simulink library "fc_vt_lib"  (Simulink 4.00)
undefined symbols (not defined in the file or in its folder): amb_tmp, compressor_mass_flow_map, compressor_pressure_map, compressor_temperature_rise_map, fc_air_comp_scale, fc_allowable_temp_rise, fc_cathode_pressure_drop, fc_cell_area, fc_cell_num, fc_comp_adeff_max, fc_comp_elec_eff, fc_comp_max_tmp, fc_comp_slpm_air_max, fc_comp_spd_max, fc_comp_voleff_max, fc_condenser_fan_flowrate, fc_condenser_fan_num, fc_condenser_fan_pwr_map, fc_condenser_frontal_area, fc_condenser_scale, fc_coolant_pump_flow_map, fc_coolant_pump_pwr_map, fc_cp_air, fc_cp_h2o_l, fc_cp_stack, fc_fuel_lhv, fc_k_air, fc_max_cathode_inlet_pressure, fc_min_cathode_inlet_pressure, fc_min_cell_volts, fc_min_sys_pwr_req, fc_min_temp_for_heat_rejection, fc_mw_air, fc_mw_h2, fc_mw_h20, fc_o2_percent, fc_p_amb, fc_polar_param_concentration, fc_polar_param_ohmic, fc_polar_param_ohmic_temp, fc_polar_param_ref_temp, fc_polar_param_tafel, fc_polar_param_temperature, fc_polar_param_voc, fc_radiator_bypass_delta_t, fc_radiator_fan_flowrate, fc_radiator_fan_num, fc_radiator_fan_pwr_map, fc_radiator_frontal_area, fc_radiator_no_fan_flowrate, fc_radiator_scale, fc_radiator_spd_ratio_fan_off, fc_radiator_spd_ratio_fan_on, fc_radiator_veh_spd_map, fc_reference_temperature, fc_rh_amb, fc_stack_i_map, fc_stack_pres_cor_map, fc_stack_pres_map, fc_stack_stoich_air_map ... (+10)
libraries: fc_vt_lib x54, simulink3 x9
(part 3 of 3)

== system fc_vt_lib/Main Loop/ambient pressure, temperature & density calc (atm) ==
  note: Ambient
      | temperature [K]
  elevation : Inport  Port=1  LatchInput=off
  Constant1 : Constant  Value=288.15
  Constant2 : Constant  Value=288.15
  Constant3 : Constant  Value=0.0065
  Math Function2 : Math  Operator=pow  OutputSignalType=auto
  Pressure [mbar] : Product  Inputs=*/  Multiplication=Element-wise(.*)  SaturateOnIntegerOverflow=on
  Pressure1 : Constant  Value=-5.255877
  Pressure2 : Constant  Value=0.3483677
  Pressure5 : Constant  Value=1013.25
  Pressure6 : Constant  Value=1013.25
  Product : Product  Inputs=2  Multiplication=Element-wise(.*)  SaturateOnIntegerOverflow=on
  Product2 : Product  Inputs=*/  Multiplication=Element-wise(.*)  SaturateOnIntegerOverflow=on
  Product3 : Product  Inputs=2  Multiplication=Element-wise(.*)  SaturateOnIntegerOverflow=on
  Product5 : Product  Inputs=*/  Multiplication=Element-wise(.*)  SaturateOnIntegerOverflow=on
  Product6 : Product  Inputs=2  Multiplication=Element-wise(.*)  SaturateOnIntegerOverflow=on
  Sum1 : Sum  Inputs=-+  SaturateOnIntegerOverflow=on
  "Ambient pressure [atm] " : Outport  Port=1
  Air density [kg/m3] : Outport  Port=2
  wires:
  Constant1/1 -> Sum1/2
  Pressure2/1 -> Product3/1
  elevation/1 -> Product/1
  Constant3/1 -> Product/2
  Product/1 -> Sum1/1
  Sum1/1 -> Product5/2, Product2/2
  Constant2/1 -> Product5/1
  Product5/1 -> Math Function2/1
  Pressure1/1 -> Math Function2/2
  Math Function2/1 -> Product6/1
  Pressure5/1 -> Product6/2
  Product6/1 -> Pressure [mbar]/1
  Pressure6/1 -> Pressure [mbar]/2
  Pressure [mbar]/1 -> "Ambient pressure [atm] "/1, Product2/1
  Product2/1 -> Product3/2
  Product3/1 -> Air density [kg/m3]/1

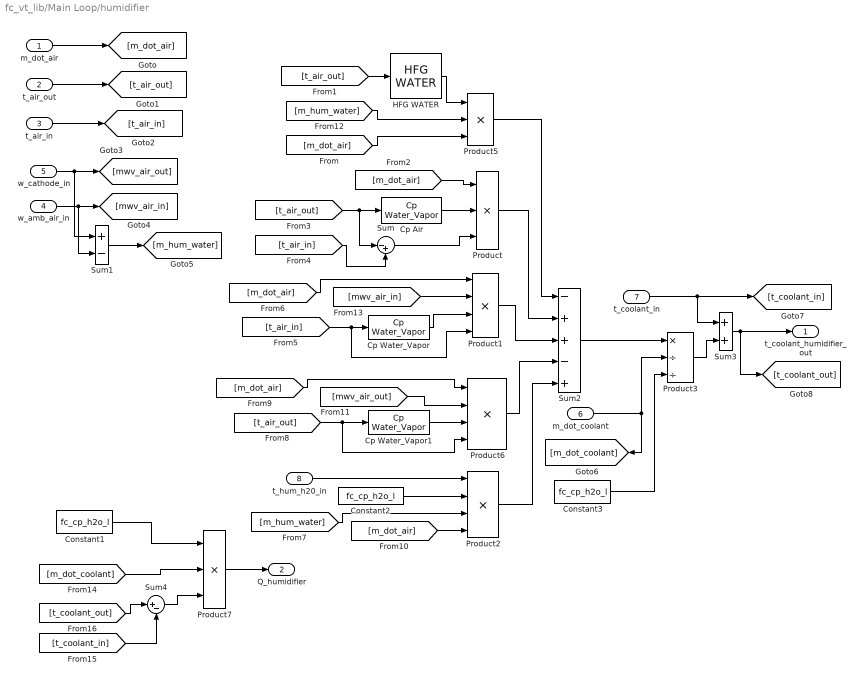
== system fc_vt_lib/Main Loop/humidifier ==
  m_dot_air : Inport  Port=1  LatchInput=off
  t_air_out : Inport  Port=2  LatchInput=off
  t_air_in : Inport  Port=3  LatchInput=off
  w_amb_air_in : Inport  Port=4  LatchInput=off
  w_cathode_in : Inport  Port=5  LatchInput=off
  m_dot_coolant : Inport  Port=6  LatchInput=off
  t_coolant_in : Inport  Port=7  LatchInput=off
  t_hum_h20_in : Inport  Port=8  LatchInput=off
  Constant1 : Constant  Value=fc_cp_h2o_l
  Constant2 : Constant  Value=fc_cp_h2o_l
  Constant3 : Constant  Value=fc_cp_h2o_l
  Cp Air : fc_vt_lib/Cp Water_Vapor
      settings: RTWFcnNameOpts=Auto  RTWFileNameOpts=Auto
  Cp Water_Vapor : fc_vt_lib/Cp Water_Vapor
      settings: RTWFcnNameOpts=Auto  RTWFileNameOpts=Auto
  Cp Water_Vapor1 : fc_vt_lib/Cp Water_Vapor
      settings: RTWFcnNameOpts=Auto  RTWFileNameOpts=Auto
  HFG WATER : fc_vt_lib/HFG WATER
      settings: RTWFcnNameOpts=Auto  RTWFileNameOpts=Auto
  Product : Product  Inputs=3  Multiplication=Element-wise(.*)  SaturateOnIntegerOverflow=on
  Product1 : Product  Inputs=4  Multiplication=Element-wise(.*)  SaturateOnIntegerOverflow=on
  Product2 : Product  Inputs=4  Multiplication=Element-wise(.*)  SaturateOnIntegerOverflow=on
  Product3 : Product  Inputs=*//  Multiplication=Element-wise(.*)  SaturateOnIntegerOverflow=on
  Product5 : Product  Inputs=3  Multiplication=Element-wise(.*)  SaturateOnIntegerOverflow=on
  Product6 : Product  Inputs=4  Multiplication=Element-wise(.*)  SaturateOnIntegerOverflow=on
  Product7 : Product  Inputs=3  Multiplication=Element-wise(.*)  SaturateOnIntegerOverflow=on
  Sum : Sum  Inputs=|-+  SaturateOnIntegerOverflow=on
  Sum1 : Sum  Inputs=+-  SaturateOnIntegerOverflow=on
  Sum2 : Sum  Inputs=-++-+  SaturateOnIntegerOverflow=on
  Sum3 : Sum  Inputs=++  SaturateOnIntegerOverflow=on
  Sum4 : Sum  Inputs=|+-  SaturateOnIntegerOverflow=on
  t_coolant_humidifier_out : Outport  Port=1
  Q_humidifier : Outport  Port=2
  wires:
  [m_dot_air] -> Product2/4
  Product1/1 -> Sum2/3
  Product/1 -> Sum2/2
  Product5/1 -> Sum2/1
  [t_air_out] -> Product6/4, Cp Water_Vapor1/1
  [m_dot_air] -> Product6/1
  Cp Water_Vapor1/1 -> Product6/3
  [m_hum_water] -> Product2/3
  [m_dot_air] -> Product1/1
  [t_air_in] -> Product1/4, Cp Water_Vapor/1
  [t_air_in] -> Sum/2
  t_air_in/1 -> [t_air_in]
  [t_air_out] -> Sum/1, Cp Air/1
  [m_dot_air] -> Product/1
  [t_air_out] -> HFG WATER/1
  [m_dot_air] -> Product5/3
  t_air_out/1 -> [t_air_out]
  HFG WATER/1 -> Product5/1
  w_cathode_in/1 -> [mwv_air_out], Sum1/1
  t_hum_h20_in/1 -> Product2/1
  Constant2/1 -> Product2/2
  Cp Water_Vapor/1 -> Product1/3
  Sum3/1 -> t_coolant_humidifier_out/1, [t_coolant_out]
  Constant3/1 -> Product3/3
  Product3/1 -> Sum3/2
  t_coolant_in/1 -> Sum3/1, [t_coolant_in]
  m_dot_coolant/1 -> Product3/2, [m_dot_coolant]
  Sum2/1 -> Product3/1
  Sum/1 -> Product/3
  Cp Air/1 -> Product/2
  m_dot_air/1 -> [m_dot_air]
  [mwv_air_out] -> Product6/2
  Constant1/1 -> Product7/1
  [m_dot_coolant] -> Product7/2
  [t_coolant_out] -> Sum4/1
  [t_coolant_in] -> Sum4/2
  Sum4/1 -> Product7/3
  Product7/1 -> Q_humidifier/1
  [m_hum_water] -> Product5/2
  w_amb_air_in/1 -> [mwv_air_in], Sum1/2
  [mwv_air_in] -> Product1/2
  Sum1/1 -> [m_hum_water]
  Product6/1 -> Sum2/4
  Product2/1 -> Sum2/5

== system fc_vt_lib/Stack Operating Point Calculation/Polarization Curve ==
  temperature : Inport  Port=1  LatchInput=off
  po2 : Inport  Port=2  LatchInput=off
  current : Inport  Port=3  LatchInput=off
  Constant : Constant  Value=fc_polar_param_voc
  Constant1 : Constant  Value=fc_polar_param_tafel
  Constant2 : Constant  Value=fc_polar_param_ohmic
  Constant3 : Constant  Value=fc_polar_param_ohmic_temp
  Constant5 : Constant  Value=fc_polar_param_temperature
  Constant6 : Constant  Value=fc_polar_param_ref_temp
  Constant7 : Constant  Value=fc_polar_param_concentration
  Gain : Gain  Gain=1000  Multiplication=Element-wise(K.*u)  SaturateOnIntegerOverflow=on
  Gain1 : Gain  Gain=1/0.21  Multiplication=Element-wise(K.*u)  SaturateOnIntegerOverflow=on
  Math Function : Math  Operator=log10  OutputSignalType=auto
  Math Function2 : Math  Operator=log10  OutputSignalType=auto
  Memory : Memory  X0=0.8  InheritSampleTime=off
      settings: RTWStateStorageClass=Auto
  Product : Product  Inputs=2  Multiplication=Element-wise(.*)  SaturateOnIntegerOverflow=on
  Product1 : Product  Inputs=2  Multiplication=Element-wise(.*)  SaturateOnIntegerOverflow=on
  Product3 : Product  Inputs=3  Multiplication=Element-wise(.*)  SaturateOnIntegerOverflow=on
  Product4 : Product  Inputs=2  Multiplication=Element-wise(.*)  SaturateOnIntegerOverflow=on
  Product5 : Product  Inputs=3  Multiplication=Element-wise(.*)  SaturateOnIntegerOverflow=on
  Sum : Sum  Inputs=+--++  SaturateOnIntegerOverflow=on
  Sum1 : Sum  Inputs=|+-  SaturateOnIntegerOverflow=on
  Sum2 : Sum  Inputs=|+-  SaturateOnIntegerOverflow=on
  cell voltage : Outport  Port=1
  wires:
  Sum/1 -> Memory/1
  Memory/1 -> cell voltage/1
  Sum1/1 -> Product4/2
  Product4/1 -> Sum/3
  Constant3/1 -> Product1/1
  Product3/1 -> Sum/5
  [pc1] -> Product3/3
  Constant5/1 -> Product3/2
  Sum2/1 -> Product3/1
  Constant6/1 -> Sum2/2
  po2/1 -> Gain1/1
  Product1/1 -> Sum1/2
  temperature/1 -> Product1/2, Sum2/1
  Constant2/1 -> Sum1/1
  Product/1 -> Sum/2
  Math Function/1 -> [pc1], Product/2
  Gain/1 -> Math Function/1, Product5/1
  current/1 -> Product4/1, Gain/1
  Constant1/1 -> Product/1
  Constant/1 -> Sum/1
  Gain1/1 -> Math Function2/1
  Product5/1 -> Sum/4
  Math Function2/1 -> Product5/3
  Constant7/1 -> Product5/2

== system fc_vt_lib/Stack Operating Point Calculation -min voltage/Polarization Curve ==
  temperature : Inport  Port=1  LatchInput=off
  po2 : Inport  Port=2  LatchInput=off
  current : Inport  Port=3  LatchInput=off
  Constant : Constant  Value=fc_polar_param_voc
  Constant1 : Constant  Value=fc_polar_param_tafel
  Constant2 : Constant  Value=fc_polar_param_ohmic
  Constant3 : Constant  Value=fc_polar_param_ohmic_temp
  Constant4 : Constant  Value=fc_polar_param_concentration
  Constant5 : Constant  Value=fc_polar_param_temperature
  Constant6 : Constant  Value=fc_polar_param_ref_temp
  Gain : Gain  Gain=1000  Multiplication=Element-wise(K.*u)  SaturateOnIntegerOverflow=on
  Gain1 : Gain  Gain=1/0.21  Multiplication=Element-wise(K.*u)  SaturateOnIntegerOverflow=on
  Math Function : Math  Operator=log10  OutputSignalType=auto
  Math Function1 : Math  Operator=log10  OutputSignalType=auto
  No Memory : Subsystem
      settings: RTWFcnNameOpts=Auto  RTWFileNameOpts=Auto
      mask Display: plot([0 1],[0.5 0.5]
  Product : Product  Inputs=2  Multiplication=Element-wise(.*)  SaturateOnIntegerOverflow=on
  Product1 : Product  Inputs=2  Multiplication=Element-wise(.*)  SaturateOnIntegerOverflow=on
  Product2 : Product  Inputs=3  Multiplication=Element-wise(.*)  SaturateOnIntegerOverflow=on
  Product3 : Product  Inputs=3  Multiplication=Element-wise(.*)  SaturateOnIntegerOverflow=on
  Product4 : Product  Inputs=2  Multiplication=Element-wise(.*)  SaturateOnIntegerOverflow=on
  Sum : Sum  Inputs=+--++  SaturateOnIntegerOverflow=on
  Sum1 : Sum  Inputs=|+-  SaturateOnIntegerOverflow=on
  Sum2 : Sum  Inputs=|+-  SaturateOnIntegerOverflow=on
  cell voltage : Outport  Port=1
  wires:
  Constant/1 -> Sum/1
  Constant1/1 -> Product/1
  current/1 -> Gain/1, Product4/1
  Gain/1 -> Math Function/1, Product2/1
  Math Function/1 -> Product/2, [pc1]
  Product/1 -> Sum/2
  Constant2/1 -> Sum1/1
  temperature/1 -> Sum2/1, Product1/2
  Product1/1 -> Sum1/2
  po2/1 -> Gain1/1
  Product2/1 -> Sum/4
  Constant6/1 -> Sum2/2
  Sum2/1 -> Product3/1
  Constant5/1 -> Product3/2
  [pc1] -> Product3/3
  Product3/1 -> Sum/5
  Constant3/1 -> Product1/1
  Product4/1 -> Sum/3
  Sum1/1 -> Product4/2
  No Memory/1(Out1) -> cell voltage/1
  Sum/1 -> No Memory/1(In1)
  Math Function1/1 -> Product2/3
  Gain1/1 -> Math Function1/1
  Constant4/1 -> Product2/2

== system fc_vt_lib/VT_FUELCELL_MODEL/Subsystem ==
  In1 : Inport  Port=1  LatchInput=off
  Bus Creator : BusCreator  Inputs=34
  Demux : Demux  Outputs=34  BusSelectionMode=off
  system_characteristics : Outport  Port=1
  wires:
  Demux/30 -> Bus Creator/30  "water_balance"
  Demux/29 -> Bus Creator/29  "condenser_working_capacity"
  Demux/28 -> Bus Creator/28  "cell_voltage"
  Demux/23 -> Bus Creator/23  "mwv_anode_inlet"
  Demux/24 -> Bus Creator/24  "mwv_cathode_inlet"
  Demux/25 -> Bus Creator/25  "water_gen"
  Demux/26 -> Bus Creator/26  "mwv_cathode_outlet"
  Demux/27 -> Bus Creator/27  "condenser_recovered_water"
  Demux/1 -> Bus Creator/1  "fc_gross_power_gen"
  Demux/2 -> Bus Creator/2  "air_compressor_power"
  Demux/3 -> Bus Creator/3  "condenser_fan_power"
  Demux/4 -> Bus Creator/4  "radiator_fan_power"
  Demux/5 -> Bus Creator/5  "coolant_pump_power"
  Demux/6 -> Bus Creator/6  "m_dot_air"
  Demux/7 -> Bus Creator/7  "m_dot_coolant"
  Demux/8 -> Bus Creator/8  "pressure_inlet_cathode"
  Demux/9 -> Bus Creator/9  "fc_cell_current"
  Demux/10 -> Bus Creator/10  "m_dot_h2"
  Demux/11 -> Bus Creator/11  "q_gen_stack"
  Demux/12 -> Bus Creator/12  "t_stack_coolant_in"
  Demux/13 -> Bus Creator/13  "t_stack_coolant_output"
  Demux/14 -> Bus Creator/14  "t_humidifier_coolant_out"
  Demux/15 -> Bus Creator/15  "t_radiator_coolant_out"
  Demux/16 -> Bus Creator/16  "condenser_heat_to_ambient"
  Demux/17 -> Bus Creator/17  "radiator_energy_loss_ambient"
  Demux/18 -> Bus Creator/18  "stack_energy_loss_ambient"
  Demux/19 -> Bus Creator/19  "reservoir_energy_loss_ambient"
  Demux/20 -> Bus Creator/20  "air_compressor_speed"
  Demux/21 -> Bus Creator/21  "air_compressor_adiabatic_efficiency"
  Demux/22 -> Bus Creator/22  "air_compressor_volumetric_efficiency"
  In1/1 -> Demux/1
  Bus Creator/1 -> system_characteristics/1
  Demux/31 -> Bus Creator/31  "condensed_water_in_stack"
  Demux/32 -> Bus Creator/32  "m_dot_h2o_anode"
  Demux/33 -> Bus Creator/33  "m_dot_h2o_cathode"
  Demux/34 -> Bus Creator/34  "stack_heat_loads"

== system fc_vt_lib/VT_FUELCELL_MODEL/min_cell_voltage & net power gen ==
  In1 : Inport  Port=1  LatchInput=off
  Action Port : ActionPort  InitializeStates=held  ActionType=unset
  Algebraic Constraint1 : Subsystem  AncestorBlock=simulink3/Math/Algebraic Constraint  mask(Algebraic Constraint){z0=40000}
      mask prompts: z0 "Initial guess:"
      mask help: Constrains input signal f(z) to zero and outputs an algebraic state z. This block outputs the value necessary to produce a zero at the input. The output must affect the input through some feedback path. Provide an initial guess of the output to improve algebraic loop solver efficiency.
      settings: RTWFcnNameOpts=Auto  RTWFileNameOpts=Auto
      mask Help:
      | This block outputs the value necessary to produce a zero at the input. The output must affect the input through some feedback path. This allows you to specify algebraic equations for index 1 differential/algebraic systems (DAE's).
      | 
      | By default, the initial guess is zero.  You can improve the efficiency of the algebraic loop solver by providing an initial guess that is close to the solution value.
      mask Display: disp('Solve\nf(z) = 0')
  Constant1 : Constant  Value=fc_min_cell_volts
  Demux1 : Demux  Outputs=4  BusSelectionMode=off
  Fuel Cell System : fc_vt_lib/Fuel Cell System
      settings: RTWFcnNameOpts=Auto  RTWFileNameOpts=Auto
  If : If  NumInputs=2  IfExpression=u1 < u2  ShowElse=off
  Mux1 : Mux  Inputs=6
  Net_power : Subsystem  TreatAsAtomicUnit=on
      settings: RTWFcnNameOpts=Auto  RTWFileNameOpts=Auto
  Sum2 : Sum  Inputs=|+-  SaturateOnIntegerOverflow=on
  Switch : Switch  Threshold=1
  Out1 : Outport  Port=1  OutputWhenDisabled=reset  InitialOutput=[0]
  wires:
  Constant1/1 -> Sum2/1
  Sum2/1 -> Algebraic Constraint1/1(f(z))
  Algebraic Constraint1/1(z) -> Fuel Cell System/1
  Fuel Cell System/1 -> Mux1/1, If/2
  Fuel Cell System/2 -> Mux1/2
  Fuel Cell System/3 -> Sum2/2, Mux1/3
  Fuel Cell System/4 -> Mux1/4
  Fuel Cell System/5 -> Mux1/5
  Demux1/2 -> Fuel Cell System/2
  Demux1/3 -> Fuel Cell System/3
  Demux1/4 -> Fuel Cell System/4
  In1/1 -> Demux1/1, Net_power/1(In1)
  Demux1/1 -> If/1
  If/1 -> Net_power/Action
  Net_power/1(Out1) -> Switch/1
  Net_power/2(Out2) -> Switch/2
  Mux1/1 -> Switch/3
  Switch/1 -> Out1/1
  Fuel Cell System/6 -> Mux1/6

== system fc_vt_lib/VT_FUELCELL_MODEL/min_system_power ==
  In1 : Inport  Port=1  LatchInput=off
  Action Port : ActionPort  InitializeStates=held  ActionType=unset
  Constant : Constant  Value=1
  Demux1 : Demux  Outputs=4  BusSelectionMode=off
  Fuel Cell System min power : fc_vt_lib/Fuel Cell System min power
      settings: RTWFcnNameOpts=Auto  RTWFileNameOpts=Auto
  Mux1 : Mux  Inputs=6
  system_characteristics : Outport  Port=1  OutputWhenDisabled=reset  InitialOutput=0
  enabled? : Outport  Port=2  OutputWhenDisabled=reset  InitialOutput=0
  wires:
  Mux1/1 -> system_characteristics/1
  In1/1 -> Demux1/1
  Constant/1 -> enabled?/1
  Demux1/1 -> Fuel Cell System min power/1
  Demux1/2 -> Fuel Cell System min power/2
  Demux1/3 -> Fuel Cell System min power/3
  Demux1/4 -> Fuel Cell System min power/4
  Fuel Cell System min power/1 -> Mux1/1
  Fuel Cell System min power/2 -> Mux1/2
  Fuel Cell System min power/3 -> Mux1/3
  Fuel Cell System min power/4 -> Mux1/4
  Fuel Cell System min power/5 -> Mux1/5
  Fuel Cell System min power/6 -> Mux1/6

== system fc_vt_lib/Fuel Cell System min power/Main Loop/Fuel_cell_stack ==
  t_stack_previous : Inport  Port=1  LatchInput=off
  Constant2 : Constant  Value=fc_stack_UA
  Constant4 : Constant  Value=amb_tmp
  Constant5 : Constant  Value=273.15
  Gain : Gain  Gain=-1  Multiplication=Element-wise(K.*u)  SaturateOnIntegerOverflow=on
  Product1 : Product  Inputs=**/  Multiplication=Element-wise(.*)  SaturateOnIntegerOverflow=on
  Product2 : Product  Inputs=2  Multiplication=Element-wise(.*)  SaturateOnIntegerOverflow=on
  Sum : Sum  Inputs=|++  SaturateOnIntegerOverflow=on
  Sum2 : Sum  Inputs=|+-  SaturateOnIntegerOverflow=on
  Sum3 : Sum  Inputs=|++  SaturateOnIntegerOverflow=on
  Time Step : fc_vt_lib/Time Step
      settings: RTWFcnNameOpts=Auto  RTWFileNameOpts=Auto
  m*Cp : Constant  Value=fc_stack_unit_mass*fc_cell_area*fc_cell_num*fc_cp_stack
  Out1 : Outport  Port=1
  stack_energy_loss_ambient : Outport  Port=2
  wires:
  Gain/1 -> Product1/2
  [t_stack_previous] -> Sum3/1
  Product1/1 -> Sum3/2
  Sum3/1 -> Out1/1
  Time Step/1 -> Product1/1
  m*Cp/1 -> Product1/3
  Product2/1 -> Gain/1, stack_energy_loss_ambient/1
  Sum2/1 -> Product2/2
  Constant2/1 -> Product2/1
  [t_stack_previous] -> Sum2/1
  t_stack_previous/1 -> [t_stack_previous]
  Constant5/1 -> Sum/1
  Sum/1 -> Sum2/2  "[K]"
  Constant4/1 -> Sum/2

== system fc_vt_lib/Fuel Cell System min power/Main Loop/Radiator ==
  Radiator Coolant Input : Inport  Port=1  LatchInput=off
  Radiator_energy_loss_ambient : Outport  Port=1
  wires:
  Radiator Coolant Input/1 -> Radiator_energy_loss_ambient/1

== system fc_vt_lib/Fuel Cell System min power/Main Loop/humidifier ==
  t_coolant_in : Inport  Port=1  LatchInput=off
  t_coolant_humidifier_out : Outport  Port=1
  wires:
  t_coolant_in/1 -> t_coolant_humidifier_out/1

== system fc_vt_lib/Main Loop/Air Compressor Calculations/air_power ==
  note: [K]
  m_dot_air : Inport  Port=1  LatchInput=off
  eff_overall : Inport  Port=2  LatchInput=off
  pressure : Inport  Port=3  LatchInput=off
  Constant : Constant  Value=amb_tmp
  Constant1 : Constant  Value=fc_k_air
  Constant2 : Constant  Value=fc_k_air
  Constant3 : Constant  Value=1
  Constant5 : Constant  Value=1
  Constant6 : Constant  Value=fc_comp_elec_eff
  Cp Air : fc_vt_lib/Cp Water_Vapor
      settings: RTWFcnNameOpts=Auto  RTWFileNameOpts=Auto
  Math Function : Math  Operator=pow  OutputSignalType=auto
  Product : Product  Inputs=4  Multiplication=Element-wise(.*)  SaturateOnIntegerOverflow=on
  Product1 : Product  Inputs=*/  Multiplication=Element-wise(.*)  SaturateOnIntegerOverflow=on
  Product2 : Product  Inputs=*//  Multiplication=Element-wise(.*)  SaturateOnIntegerOverflow=on
  Sum : Sum  Inputs=|+-  SaturateOnIntegerOverflow=on
  Sum1 : Sum  Inputs=|+-  SaturateOnIntegerOverflow=on
  Sum2 : Sum  Inputs=|++  SaturateOnIntegerOverflow=on
  const : Constant  Value=273.15
  Out1 : Outport  Port=1
  wires:
  m_dot_air/1 -> Product/1
  Constant1/1 -> Sum/1
  Constant3/1 -> Sum/2
  Sum/1 -> Product1/1
  Constant2/1 -> Product1/2
  pressure/1 -> Math Function/1
  Product1/1 -> Math Function/2
  Constant5/1 -> Sum1/2
  Math Function/1 -> Sum1/1
  Sum1/1 -> Product/4
  Product/1 -> Product2/1
  Constant6/1 -> Product2/2
  eff_overall/1 -> Product2/3
  Product2/1 -> Out1/1
  Cp Air/1 -> Product/2
  Sum2/1 -> Cp Air/1, Product/3
  Constant/1 -> Sum2/2
  const/1 -> Sum2/1

== system fc_vt_lib/Main Loop/Air Requirement Calculation/Molecular Weight of  Inlet Air (g/mole) ==
  In1 : Inport  Port=1  LatchInput=off
  In2 : Inport  Port=2  LatchInput=off
  In3 : Inport  Port=3  LatchInput=off
  Product1 : Product  Inputs=2  Multiplication=Element-wise(.*)  SaturateOnIntegerOverflow=on
  Product2 : Product  Inputs=2  Multiplication=Element-wise(.*)  SaturateOnIntegerOverflow=on
  Sum : Sum  Inputs=+-  SaturateOnIntegerOverflow=on
  Sum1 : Sum  Inputs=++  SaturateOnIntegerOverflow=on
  constant : Constant  Value=1
  Out1 : Outport  Port=1
  wires:
  In1/1 -> Product2/1, Sum/2
  constant/1 -> Sum/1
  Sum/1 -> Product1/2
  In3/1 -> Product1/1
  Product1/1 -> Sum1/1
  Product2/1 -> Sum1/2
  In2/1 -> Product2/2
  Sum1/1 -> Out1/1

== system fc_vt_lib/Main Loop/Control Stratgegy for FC inlet cathode pressure/Limit Pressure ==
  p req : Inport  Port=1  LatchInput=off
  p amb : Inport  Port=2  LatchInput=off
  Constant : Constant  Value=compressor_pressure_map
  Constant1 : Constant  Value=compressor_pressure_map
  MinMax : MinMax  Function=min  Inputs=2
  MinMax1 : MinMax  Function=max  Inputs=1
  MinMax2 : MinMax  Function=max  Inputs=3
  MinMax3 : MinMax  Function=min  Inputs=1
  Product : Product  Inputs=2  Multiplication=Element-wise(.*)  SaturateOnIntegerOverflow=on
  Product1 : Product  Inputs=2  Multiplication=Element-wise(.*)  SaturateOnIntegerOverflow=on
  Sum2 : Sum  Inputs=++  SaturateOnIntegerOverflow=on
  dim % : Constant  Value=fc_cathode_pressure_drop
  p req  limited : Outport  Port=1
  wires:
  Constant/1 -> MinMax1/1
  Product/1 -> MinMax/2
  p req/1 -> MinMax/1
  dim %/1 -> Sum2/2
  MinMax1/1 -> Product/1
  p amb/1 -> Product/2, Sum2/1, Product1/2
  MinMax/1 -> MinMax2/1
  MinMax2/1 -> p req  limited/1
  Sum2/1 -> MinMax2/2
  Constant1/1 -> MinMax3/1
  MinMax3/1 -> Product1/1
  Product1/1 -> MinMax2/3

== system fc_vt_lib/Main Loop/Subsystem2/Enthalpy [kj/kg]  Look-Up Table (2-D) ==
  Rows : Inport  Port=1  LatchInput=off
  Cols : Inport  Port=2  LatchInput=off
  Look-Up Table (2-D) : Lookup2D  RowIndex=x  ColumnIndex=y  OutputValues=t
  Out1 : Outport  Port=1
  wires:
  Rows/1 -> Look-Up Table (2-D)/1
  Cols/1 -> Look-Up Table (2-D)/2
  Look-Up Table (2-D)/1 -> Out1/1

== system fc_vt_lib/Stack Operating Point Calculation -min voltage/Polarization Curve/No Memory ==
  In1 : Inport  Port=1  LatchInput=off
  Out1 : Outport  Port=1
  wires:
  In1/1 -> Out1/1

== system fc_vt_lib/VT_FUELCELL_MODEL/min_cell_voltage & net power gen/Algebraic Constraint1 ==
  f(z) : Inport  Port=1  LatchInput=off
  Initial Guess : InitialCondition  Value=z0
  Sum : Sum  Inputs=|++  SaturateOnIntegerOverflow=on
  z : Outport  Port=1
  wires:
  Sum/1 -> Initial Guess/1
  Initial Guess/1 -> Sum/2, z/1
  f(z)/1 -> Sum/1

== system fc_vt_lib/VT_FUELCELL_MODEL/min_cell_voltage & net power gen/Net_power ==
  In1 : Inport  Port=1  LatchInput=off
  Action Port : ActionPort  InitializeStates=held  ActionType=then
  Algebraic Constraint : Subsystem  AncestorBlock=simulink3/Math/Algebraic Constraint  mask(Algebraic Constraint){z0=20000}
      mask prompts: z0 "Initial guess:"
      mask help: Constrains input signal f(z) to zero and outputs an algebraic state z. This block outputs the value necessary to produce a zero at the input. The output must affect the input through some feedback path. Provide an initial guess of the output to improve algebraic loop solver efficiency.
      settings: RTWFcnNameOpts=Auto  RTWFileNameOpts=Auto
      mask Help:
      | This block outputs the value necessary to produce a zero at the input. The output must affect the input through some feedback path. This allows you to specify algebraic equations for index 1 differential/algebraic systems (DAE's).
      | 
      | By default, the initial guess is zero.  You can improve the efficiency of the algebraic loop solver by providing an initial guess that is close to the solution value.
      mask Display: disp('Solve\nf(z) = 0')
  Constant : Constant  Value=1
  Demux1 : Demux  Outputs=4  BusSelectionMode=off
  Fuel Cell System : fc_vt_lib/Fuel Cell System
      settings: RTWFcnNameOpts=Auto  RTWFileNameOpts=Auto
  Mux : Mux  Inputs=6
  Sum : Sum  Inputs=|+-  SaturateOnIntegerOverflow=on
  Out1 : Outport  Port=1  OutputWhenDisabled=reset  InitialOutput=0
  Out2 : Outport  Port=2  OutputWhenDisabled=reset  InitialOutput=0
  wires:
  Algebraic Constraint/1(z) -> Fuel Cell System/1
  Sum/1 -> Algebraic Constraint/1(f(z))
  Mux/1 -> Out1/1
  In1/1 -> Demux1/1
  Demux1/1 -> Sum/1
  Demux1/2 -> Fuel Cell System/2
  Demux1/3 -> Fuel Cell System/3
  Demux1/4 -> Fuel Cell System/4
  Fuel Cell System/1 -> Mux/1, Sum/2
  Fuel Cell System/2 -> Mux/2
  Fuel Cell System/3 -> Mux/3
  Fuel Cell System/4 -> Mux/4
  Fuel Cell System/5 -> Mux/5
  Constant/1 -> Out2/1
  Fuel Cell System/6 -> Mux/6

== system fc_vt_lib/VT_FUELCELL_MODEL/min_cell_voltage & net power gen/Net_power/Algebraic Constraint ==
  f(z) : Inport  Port=1  LatchInput=off
  Initial Guess : InitialCondition  Value=z0
  Sum : Sum  Inputs=|++  SaturateOnIntegerOverflow=on
  z : Outport  Port=1
  wires:
  Sum/1 -> Initial Guess/1
  Initial Guess/1 -> Sum/2, z/1
  f(z)/1 -> Sum/1
